simulink model "FilterModel"  (R2023a)
settings: Solver=VariableStepAuto  StartTime=0.0  StopTime=10.0  RelTol=1e-3
undefined symbols (not defined in the file): fdesignblkfcn, gcbh
libraries: dspvision x1
settings Model: Creator=wcpth  LastModifiedBy=wcpth

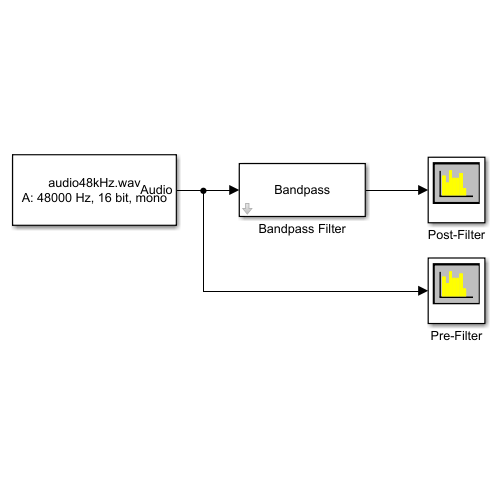
[thumbnail: Simulink's stored preview of the top-level diagram]
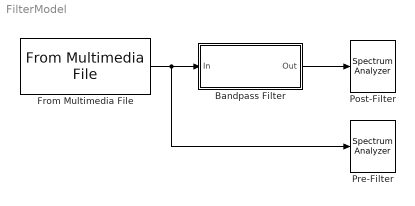
== system FilterModel ==
  Bandpass Filter : Subsystem  DialogController=fdesignblkfcn  InitFcn=fdesignblkfcn(gcbh, {'InitFcn'});  mask(Bandpass Filter){}
      mask help: dsp:DSPFilterDesignBlockDialog:BandpassFdesign_MaskDesc
      settings: CopyFcn=fdesignblkfcn(gcbh, {'CopyFcn'});
      mask Help: helpview(mapfilelocation('dsp'), 'dspbandpassfilter');
      mask Display: disp('Bandpass');
  From Multimedia File : dspvision/From Multimedia File  inputFilename=C:\Program Files\MATLAB\R2023a\toolbox\dsp\samples\audio48kHz.wav  readRange=[1 Inf]  loop=on  numPlays=1  outputStreams=Audio only  videoDataType=single  audioDataType=single  inheritSampleTime=on  userDefinedSampleTime=1/30  noAudioOutput=off  isIntensityVideo=off  fourcc=RGB  colorVideoFormat=Separate color signals  outputEOF=off  dataOrg=Column-major  audioFrameSize=1024  computeAudioFrameSize=off  outSamplingMode=Sample based
      settings: LibrarySourceBlock=audiosources/From Multimedia File
  Post-Filter : SpectrumAnalyzer  WindowPosition=[199.000000,16.000000,800.000000,500.000000,]  ScopeFrameLocation=window  SampleRateSource=Property  SampleRate=44.1e3  PlotAsTwoSidedSpectrum=off  FrequencyScale=Log  FrequencySpan=Start and stop frequencies  StartFrequency=20  StopFrequency=20e3  YLimits=[-190.76516535,18.49492481]  ColorLimits=[-20 80]  DefaultConfigurationName=spbscopes.SpectrumAnalyzerBlockCfg  IsFrequencyInputMode=0  FrequencyVectorPort=0  FrequencyVectorFromPort=0  FrequencyInputRBWPort=0  FrequencyInputRBWFromPort=0
  Pre-Filter : SpectrumAnalyzer  WindowPosition=[198.000000,487.000000,800.000000,500.000000,]  ScopeFrameLocation=window  SampleRateSource=Property  SampleRate=44.1e3  PlotAsTwoSidedSpectrum=off  FrequencyScale=Log  FrequencySpan=Start and stop frequencies  StartFrequency=20  StopFrequency=20e3  YLimits=[-96.76751977,15.48660125]  ColorLimits=[-20 80]  DefaultConfigurationName=spbscopes.SpectrumAnalyzerBlockCfg  IsFrequencyInputMode=0  FrequencyVectorPort=0  FrequencyVectorFromPort=0  FrequencyInputRBWPort=0  FrequencyInputRBWFromPort=0
  wires:
  From Multimedia File/1 -> Pre-Filter/1, Bandpass Filter/1(In)
  Bandpass Filter/1(Out) -> Post-Filter/1

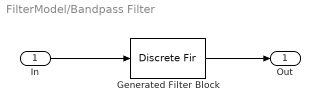
== system FilterModel/Bandpass Filter ==
  In : Inport
  Generated Filter Block : DiscreteFir  Tag=BlockMethodSubSystem  FilterStructure=Direct form symmetric  Coefficients=[-0.000524869012009213033 -0.00176959965478555603 -7.94174521698447683e-05 -0.00171105640476499916 -0.00207879238233143289 -0.000118141176326076332 -0.00438763941485114609 -0.00165397464965996027 -0.00197115773326863837 -0.00789762346591525374 0.000115874091345746162 -0.00780163204307526836 -0.00908259328672361525 0.000965742533893227165 -0.0175678643363080776 -0.00434108823623174152 -0.00451084358176348683 -0.0261267803378019518 0.0059410519837388839 -0.021335878691210914 -0.0236780648558814824 0.0139747556183038319 -0.0489686669285182147 0.000742816809324767778 0.00379690515611978696 -0.0790165169787151872 0.0636239062400671407 -0.0657944769441475424 -0.0987636679456948552 0.568467792092944957 0.568467792092944957 -0.0987636679456948552 -0.0657944769441475424 0.0636239062400671407 -0.0790165169787151872 0.00379690515611978696 0.000742816809324767778 -0.0489686669285182147 0.0139747556183038319 -0.0236780648558814824 -0.021335878691210914 0.0059410519837388839 -0.0261267803378019518 -0.00451084358176348683 -0.00434108823623174152 -0.0175678643363080776 0.000965742533893227165 -0.00908259328672361525 -0.00780163204307526836 0.000115874091345746162 -0.00789762346591525374 -0.00197115773326863837 -0.00165397464965996027 -0.00438763941485114609 -0.000118141176326076332 -0.00207879238233143289 -0.00171105640476499916 -7.94174521698447683e-05 -0.00176959965478555603 -0.000524869012009213033]  InputProcessing=Columns as channels (frame based)
  Out : Outport  VectorParamsAs1DForOutWhenUnconnected=off
  wires:
  In/1 -> Generated Filter Block/1
  Generated Filter Block/1 -> Out/1
